simulink model "irobotcomunicationWIFI"  (Simulink 7.0)
settings: Solver=FixedStepDiscrete  StartTime=0.0  StopTime=inf  FixedStep=0.1  RelTol=1e-3
libraries: nps_srllib x2, vrlib x1, utility x1
settings Model: Creator=tdlehman  LastModifiedBy=root  ExtModeAutoUpdateStatusClock=off
settings OptimizationCC: LocalBlockOutputs=off
settings DebuggingCC: AlgebraicLoopMsg=none  MultiTaskCondExecSysMsg=warning
settings RTWCC: SystemTargetFile=rtai.tlc  GenCodeOnly=on  TemplateMakefile=rtai.tmf  Description=Linux RTAI Real-Time Target  ProcessScript=rtai_make_rtw_hook  CustomInclude=./lqry/lqry
settings RTWCC: CustomSource=|
  | balgbk.o d1nrm.o dgefam.o drot.o dswap.o gradbk.o lineq.o mlineq.o mqfwo.o mulb.o
  | orthes.o qzval.o rinv.o scalbk.o symslv.o balgen.o daxpy.o dgeslm.o dscal.o exchqz.o
  | gradeq.o lypcnd.o mmul.o mscale.o mulwoa.o ortran.o reduce.o rotc.o scaleg.o trnata.o
  | cmprs.o ddot.o dnrm2.o dstslv.o fbgain.o hqrort.o lypdsd.o mqfa.o msub.o newt.o qzhesw.o
  | resid.o rotr.o sepest.o trnatb.o creg.o dgecom.o drotg.o dsvdc.o giv.o madd.o mqf.o
  | mula.o order.o qzitw.o ricsol.o save.o symprd.o xty.o
settings STFCustomTargetCC: GenFloatMathFcnCalls=ANSI_C  ModelReferenceCompliant=off  MatFileLogging=on  SystemTargetFile=rtai.tlc

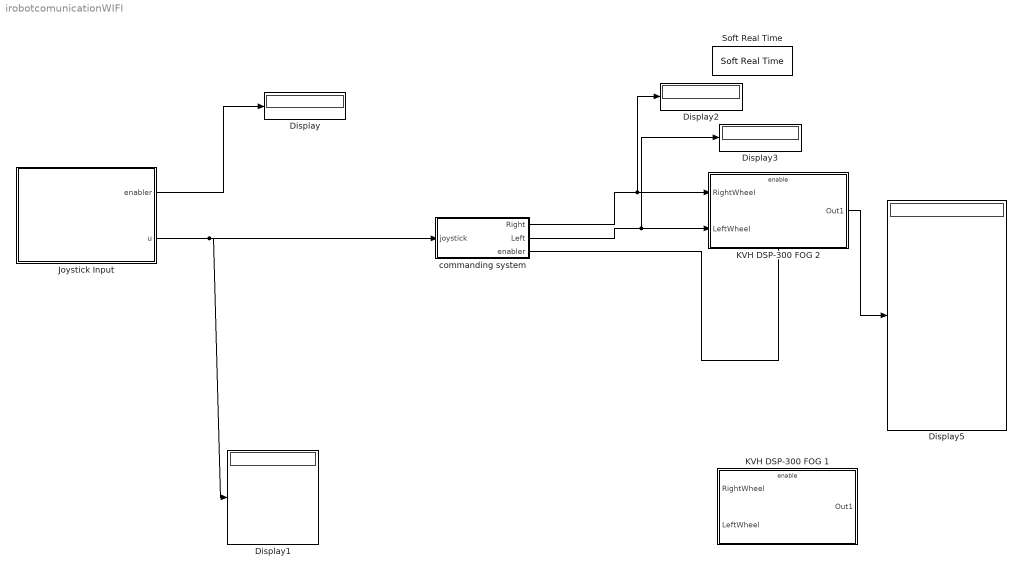
== system irobotcomunicationWIFI ==
  Display{,1..3,5} (5 alike) : Display
  Joystick Input : Subsystem
  KVH DSP-300 FOG 1 : Subsystem  mask(EZServo){port=COM1, baudrate=57600, databit=8, stopbit=1, parity=None, samptime=0.1}
      mask prompts: baudrate "Baud rate:"; databit "Number of data bits:"; stopbit "Number of stop bits:"; samptime "Sample Time:"
      mask help:
      | iRobot Create
      | (Alessio Grompone)
      |
      | Select the following options for standard use:
      |
      | 57600 bps, 8 Data Bits, 1 Stop Bit, No Parity, No Protocol
      mask StyleString: popup(COM1|COM2|COM3|COM4|COM5|COM6|COM7|COM8),popup(115200|57600|38400|19200|9600|4800|2400|1200|300|110),popup(8|7|6|5),popup(1|2),popup(None|Odd|Even),edit
      mask Display:
      | disp('iRobot \n Create UDP');
      | 
      | 
      | 
      | port_label('input',1,'Right Vel')
      | port_label('input',2,'Left Vel')
  KVH DSP-300 FOG 2 : Subsystem  mask(EZServo){port=COM1, baudrate=57600, databit=8, stopbit=1, parity=None, samptime=0.1}
      mask prompts: baudrate "Baud rate:"; databit "Number of data bits:"; stopbit "Number of stop bits:"; samptime "Sample Time:"
      mask help:
      | iRobot Create
      | (Alessio Grompone)
      |
      | Select the following options for standard use:
      |
      | 57600 bps, 8 Data Bits, 1 Stop Bit, No Parity, No Protocol
      mask StyleString: popup(COM1|COM2|COM3|COM4|COM5|COM6|COM7|COM8),popup(115200|57600|38400|19200|9600|4800|2400|1200|300|110),popup(8|7|6|5),popup(1|2),popup(None|Odd|Even),edit
      mask Display:
      | disp('iRobot \n Create');
      | 
      | 
      | 
      | port_label('input',1,'Right Vel')
      | port_label('input',2,'Left Vel')
  Soft Real Time : utility/Soft Real Time  x=1
  commanding system : Subsystem
  wires:
  Joystick Input/2(u) -> Display1/1, commanding system/1(joystick)
  Joystick Input/1(enabler) -> Display/1
  commanding system/3(enabler) -> KVH DSP-300 FOG 2/Enable
  commanding system/1(Right) -> KVH DSP-300 FOG 2/1(RightWheel), Display2/1
  commanding system/2(Left) -> KVH DSP-300 FOG 2/2(LeftWheel), Display3/1
  KVH DSP-300 FOG 2/1(Out1) -> Display5/1

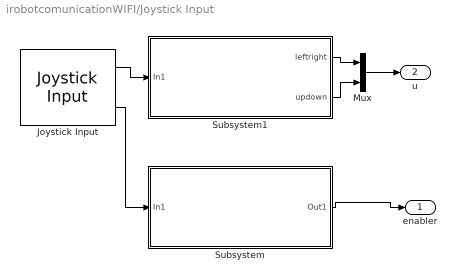
== system irobotcomunicationWIFI/Joystick Input ==
  Joystick Input : vrlib/Joystick Input  joyid=1  adjustports=on  forcefeed=off
  Mux : Mux  Inputs=2
  Subsystem : Subsystem
  Subsystem1 : Subsystem
  enabler : Outport  OutDataType=sfix(16)  OutScaling=2^0
  u : Outport  Port=2  OutDataType=sfix(16)  OutScaling=2^0
  wires:
  Joystick Input/1 -> Subsystem1/1(In1)
  Joystick Input/2 -> Subsystem/1(In1)
  Subsystem/1(Out1) -> enabler/1
  Mux/1 -> u/1
  Subsystem1/1(leftright) -> Mux/1
  Subsystem1/2(updown) -> Mux/2

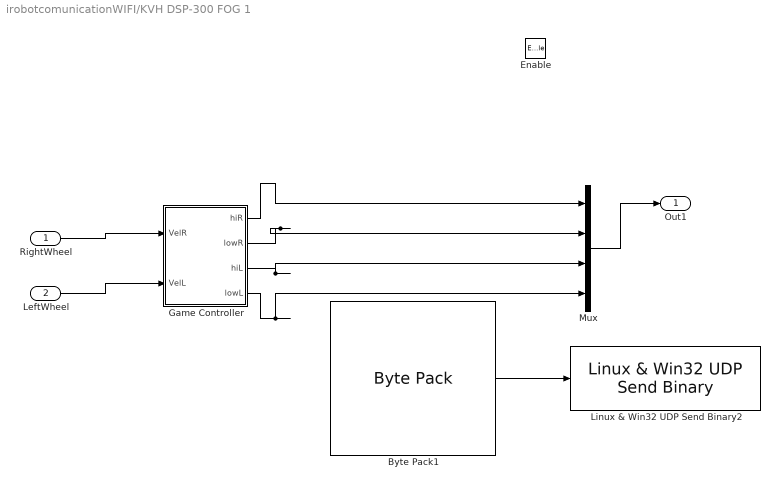
== system irobotcomunicationWIFI/KVH DSP-300 FOG 1 ==
  RightWheel : Inport  OutDataType=sfix(16)  OutScaling=2^0
  LeftWheel : Inport  Port=2  OutDataType=sfix(16)  OutScaling=2^0
  Enable : EnablePort
  Byte Pack1 : nps_srllib/UDP Comms/Byte Pack  datatypes={'double';'double';'double';'double'}  byteAlign=1
  Game Controller : Stateflow chart
  Linux & Win32 UDP Send Binary2 : nps_srllib/UDP Comms/Linux & Win32 UDP Send Binary  ipAddress=170.160.1.101  ipPort=0000  localPort=-1  sampletime=0.02
  Mux : Mux
  Out1 : Outport  OutDataType=sfix(16)  OutScaling=2^0
  wires:
  Mux/1 -> Out1/1
  LeftWheel/1 -> Game Controller/2(VelL)
  RightWheel/1 -> Game Controller/1(VelR)
  Game Controller/4(lowL) -> Mux/4
  Game Controller/3(hiL) -> Mux/3
  Game Controller/2(lowR) -> Mux/2
  Game Controller/1(hiR) -> Mux/1
  Byte Pack1/1 -> Linux & Win32 UDP Send Binary2/1

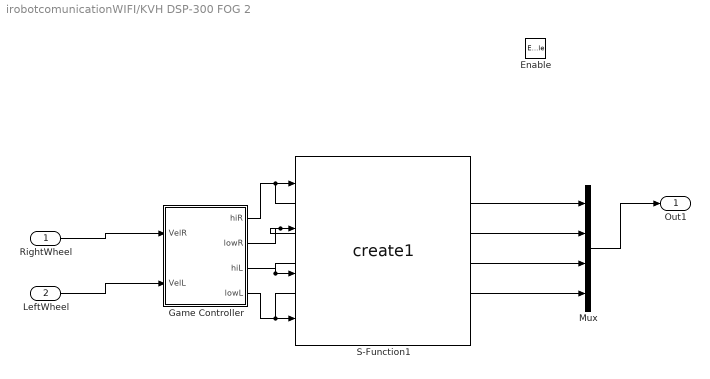
== system irobotcomunicationWIFI/KVH DSP-300 FOG 2 ==
  RightWheel : Inport  OutDataType=sfix(16)  OutScaling=2^0
  LeftWheel : Inport  Port=2  OutDataType=sfix(16)  OutScaling=2^0
  Enable : EnablePort
  Game Controller : Stateflow chart
  Mux : Mux
  S-Function1 : S-Function  FunctionName=create1  Parameters=port, baudrate, databit, stopbit, parity, samptime
  Out1 : Outport  OutDataType=sfix(16)  OutScaling=2^0
  wires:
  Game Controller/1(hiR) -> S-Function1/1, Mux/1
  Game Controller/2(lowR) -> S-Function1/2, Mux/2
  Game Controller/3(hiL) -> S-Function1/3, Mux/3
  Game Controller/4(lowL) -> S-Function1/4, Mux/4
  RightWheel/1 -> Game Controller/1(VelR)
  LeftWheel/1 -> Game Controller/2(VelL)
  Mux/1 -> Out1/1

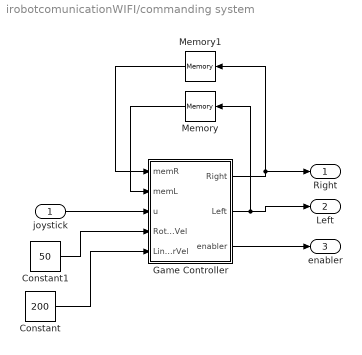
== system irobotcomunicationWIFI/commanding system ==
  joystick : Inport  OutDataType=sfix(16)  OutScaling=2^0
  Constant : Constant  Value=200  OutDataType=sfix(16)  OutScaling=2^0
  Constant1 : Constant  Value=50  OutDataType=sfix(16)  OutScaling=2^0
  Game Controller : Stateflow chart
  Memory : Memory  Orientation=left
  Memory1 : Memory  Orientation=left
  Right : Outport  OutDataType=sfix(16)  OutScaling=2^0
  Left : Outport  Port=2  OutDataType=sfix(16)  OutScaling=2^0
  enabler : Outport  Port=3  OutDataType=sfix(16)  OutScaling=2^0
  wires:
  joystick/1 -> Game Controller/3(u)
  Game Controller/1(Right) -> Memory1/1, Right/1
  Game Controller/2(Left) -> Memory/1, Left/1
  Game Controller/3(enabler) -> enabler/1
  Memory1/1 -> Game Controller/1(memR)
  Memory/1 -> Game Controller/2(memL)
  Constant/1 -> Game Controller/5(LinearVel)
  Constant1/1 -> Game Controller/4(RotationVel)

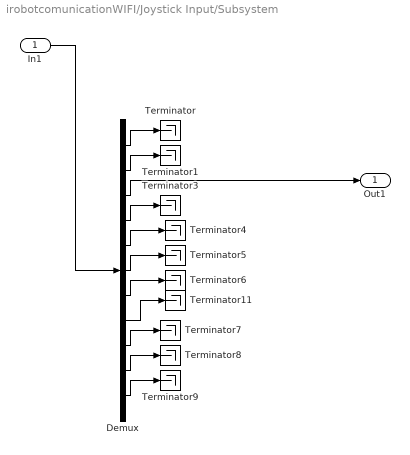
== system irobotcomunicationWIFI/Joystick Input/Subsystem ==
  In1 : Inport  OutDataType=sfix(16)  OutScaling=2^0
  Demux : Demux  Outputs=11
  Terminator{,1,3..9,11} (10 alike) : Terminator
  Out1 : Outport  OutDataType=sfix(16)  OutScaling=2^0
  wires:
  In1/1 -> Demux/1
  Demux/1 -> Terminator/1
  Demux/2 -> Terminator1/1
  Demux/3 -> Out1/1
  Demux/4 -> Terminator3/1
  Demux/5 -> Terminator4/1
  Demux/9 -> Terminator7/1
  Demux/10 -> Terminator8/1
  Demux/11 -> Terminator9/1
  Demux/6 -> Terminator5/1
  Demux/7 -> Terminator6/1
  Demux/8 -> Terminator11/1

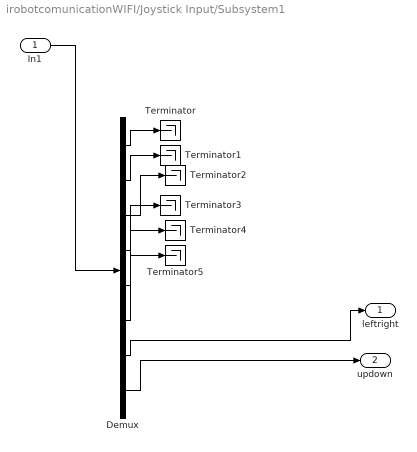
== system irobotcomunicationWIFI/Joystick Input/Subsystem1 ==
  In1 : Inport  OutDataType=sfix(16)  OutScaling=2^0
  Demux : Demux  Outputs=8
  Terminator{,1..5} (6 alike) : Terminator
  leftright : Outport  OutDataType=sfix(16)  OutScaling=2^0
  updown : Outport  Port=2  OutDataType=sfix(16)  OutScaling=2^0
  wires:
  Demux/8 -> updown/1
  Demux/7 -> leftright/1
  Demux/6 -> Terminator5/1
  Demux/5 -> Terminator4/1
  Demux/4 -> Terminator3/1
  Demux/2 -> Terminator1/1
  Demux/1 -> Terminator/1
  In1/1 -> Demux/1
  Demux/3 -> Terminator2/1

== matlab function commanding system/Game Controller ==
  data: memR input inherited; memL input inherited; u input inherited; RotationVel input inherited; LinearVel input inherited; Right output inherited; Left output inherited; enabler output inherited
function [Right,Left,enabler] = fcn(memR,memL,u,RotationVel,LinearVel)
% This block supports the Embedded MATLAB subset.
% See the help menu for details. 


if u(1)==-1; %turn right
Right=-RotationVel;
Left=RotationVel;
elseif u(1)==1;%turn left   
Right=RotationVel;
Left=-RotationVel;
else
Right=0;
Left=0;  
end


    
if u(2)==1; %backwards
Right=-LinearVel+Right;
Left=-LinearVel+Left;
elseif u(2)==-1;%forward   
Right=LinearVel+Right;
Left=LinearVel+Left;
else %stop   
Right=Right;
Left=Left;
end 

%Enabler for the S-Function

if memR==Right && memL==Left
    enabler = 0;
else
    enabler=1;
end

== matlab function KVH DSP-300 FOG 2/Game Controller ==
  data: VelR input inherited; VelL input inherited; hiR output inherited; lowR output inherited; hiL output inherited; lowL output inherited
function [hiR,lowR,hiL,lowL] = fcn(VelR,VelL)
% Alessio Grompone january 2014
% Spacecraft Robotics Laboratory, Naval Postgraduate School

%Converts Wheels velocities first to hex then to two decimals as required by iRobot Create

%Right Wheel Conversion


if VelR>0
    %decimal to numeric hex vector
    A=zeros(4,1);
    B=zeros(4,1);
    d=VelR;
    i=1;
    while d>16
        A(i)=rem(d,16);
        d=floor(d/16);
        i=i+1;
    end
    A(i)=d; %inverted numeric hex vector
    l=size(A);
    n=l(1)+1;
    for z=1:4
        B(z)=A(n-z);
    end
    %numeric hex vector to 2 decimal values
    hiR=B(1)*16+B(2);
    lowR=B(3)*16+B(4);
elseif VelR<0
    uneg=VelR+2^16;
    A=zeros(4,1);
    B=zeros(4,1);
    d=uneg;
    i=1;
    while d>16
        A(i)=rem(d,16);
        d=floor(d/16);
        i=i+1;
    end
    A(i)=d; %inverted numeric hex vector
    l=size(A);
    n=l(1);
    for z=0:n-1
        B(z+1)=A(n-z);
    end
    %numeric hex vector to 2 decimal values
    hiR=B(1)*16+B(2);
    lowR=B(3)*16+B(4);
else
    uneg=VelR+2^16;
    A=zeros(4,1);
    B=zeros(4,1);
    d=uneg;
    i=1;
    hiR=0;
    lowR=0;  
end

if VelL>0
    %decimal to numeric hex vector
    Al=zeros(4,1);
    Bl=zeros(4,1);
    dl=VelL;
    il=1;
    while dl>16
        Al(il)=rem(dl,16);
        dl=floor(dl/16);
        il=il+1;
    end
    Al(il)=dl; %inverted numeric hex vector
    ll=size(Al);
    nl=ll(1)+1;
    for zl=1:4
        Bl(zl)=Al(nl-zl);
    end
    %numeric hex vector to 2 decimal values
    hiL=Bl(1)*16+Bl(2);
    lowL=Bl(3)*16+Bl(4);
elseif VelL<0
    unegl=VelL+2^16;
    Al=zeros(4,1);
    Bl=zeros(4,1);
    dl=unegl;
    il=1;
    while dl>16
        Al(il)=rem(dl,16);
        dl=floor(dl/16);
        il=il+1;
    end
    Al(il)=dl; %inverted numeric hex vector
    ll=size(Al);
    nl=ll(1);
    for zl=0:nl-1
        Bl(zl+1)=Al(nl-zl);
    end
    %numeric hex vector to 2 decimal values
    hiL=Bl(1)*16+Bl(2);
    lowL=Bl(3)*16+Bl(4);
else
    unegl=VelL+2^16;
    Al=zeros(4,1);
    Bl=zeros(4,1);
    dl=unegl;
    il=1;
    hiL=0;
    lowL=0;
end

== matlab function KVH DSP-300 FOG 1/Game Controller ==
  data: VelR input inherited; VelL input inherited; hiR output inherited; lowR output inherited; hiL output inherited; lowL output inherited
function [hiR,lowR,hiL,lowL] = fcn(VelR,VelL)
% Alessio Grompone january 2014
% Spacecraft Robotics Laboratory, Naval Postgraduate School

%Converts Wheels velocities first to hex then to two decimals as required by iRobot Create

%Right Wheel Conversion


if VelR>0
    %decimal to numeric hex vector
    A=zeros(4,1);
    B=zeros(4,1);
    d=VelR;
    i=1;
    while d>16
        A(i)=rem(d,16);
        d=floor(d/16);
        i=i+1;
    end
    A(i)=d; %inverted numeric hex vector
    l=size(A);
    n=l(1)+1;
    for z=1:4
        B(z)=A(n-z);
    end
    %numeric hex vector to 2 decimal values
    hiR=B(1)*16+B(2);
    lowR=B(3)*16+B(4);
elseif VelR<0
    uneg=VelR+2^16;
    A=zeros(4,1);
    B=zeros(4,1);
    d=uneg;
    i=1;
    while d>16
        A(i)=rem(d,16);
        d=floor(d/16);
        i=i+1;
    end
    A(i)=d; %inverted numeric hex vector
    l=size(A);
    n=l(1);
    for z=0:n-1
        B(z+1)=A(n-z);
    end
    %numeric hex vector to 2 decimal values
    hiR=B(1)*16+B(2);
    lowR=B(3)*16+B(4);
else
    uneg=VelR+2^16;
    A=zeros(4,1);
    B=zeros(4,1);
    d=uneg;
    i=1;
    hiR=0;
    lowR=0;  
end

if VelL>0
    %decimal to numeric hex vector
    Al=zeros(4,1);
    Bl=zeros(4,1);
    dl=VelL;
    il=1;
    while dl>16
        Al(il)=rem(dl,16);
        dl=floor(dl/16);
        il=il+1;
    end
    Al(il)=dl; %inverted numeric hex vector
    ll=size(Al);
    nl=ll(1)+1;
    for zl=1:4
        Bl(zl)=Al(nl-zl);
    end
    %numeric hex vector to 2 decimal values
    hiL=Bl(1)*16+Bl(2);
    lowL=Bl(3)*16+Bl(4);
elseif VelL<0
    unegl=VelL+2^16;
    Al=zeros(4,1);
    Bl=zeros(4,1);
    dl=unegl;
    il=1;
    while dl>16
        Al(il)=rem(dl,16);
        dl=floor(dl/16);
        il=il+1;
    end
    Al(il)=dl; %inverted numeric hex vector
    ll=size(Al);
    nl=ll(1);
    for zl=0:nl-1
        Bl(zl+1)=Al(nl-zl);
    end
    %numeric hex vector to 2 decimal values
    hiL=Bl(1)*16+Bl(2);
    lowL=Bl(3)*16+Bl(4);
else
    unegl=VelL+2^16;
    Al=zeros(4,1);
    Bl=zeros(4,1);
    dl=unegl;
    il=1;
    hiL=0;
    lowL=0;
end
